simulink subsystem "LowLevelControler"  (R2022b)
settings: Solver=VariableStepAuto  StartTime=0.0  StopTime=10.0  RelTol=1e-3
settings Model: Creator=ПК  LastModifiedBy=ycheb
settings OptimizationCC: ReuseModelBlockBuffer=on

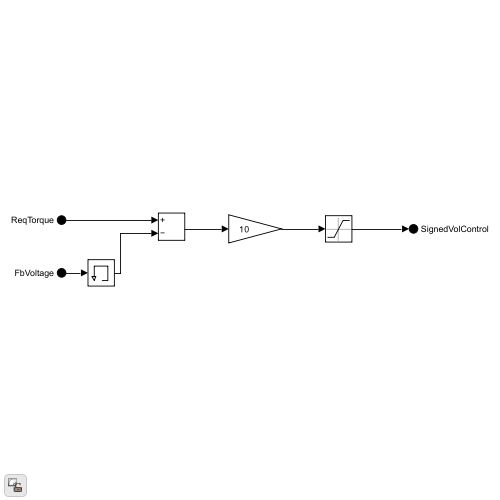
[thumbnail: Simulink's stored preview of the top-level diagram]
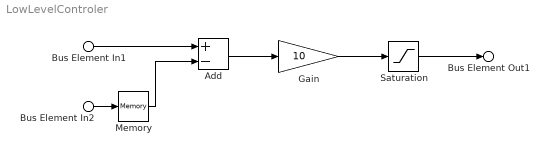
== system LowLevelControler ==
  Bus Element In1 : Inport  PortName=ReqTorque
  Bus Element In2 : Inport  Port=2  PortName=FbVoltage
  Add : Sum  Inputs=+-
  Gain : Gain  Gain=10
  Memory : Memory
  Saturation : Saturate  UpperLimit=3.3  LowerLimit=0
  Bus Element Out1 : Outport  PortName=SignedVolControl
  wires:
  Bus Element In1/1 -> Add/1
  Bus Element In2/1 -> Memory/1
  Saturation/1 -> Bus Element Out1/1
  Memory/1 -> Add/2
  Add/1 -> Gain/1
  Gain/1 -> Saturation/1
